simulink model "pure_pursuit"  (R2015b)
settings: Solver=FixedStepDiscrete  StartTime=0.0  StopTime=3  FixedStep=0.01  RelTol=1e-3
settings Model: Creator=castiel_liu  LastModifiedBy=castiel_liu

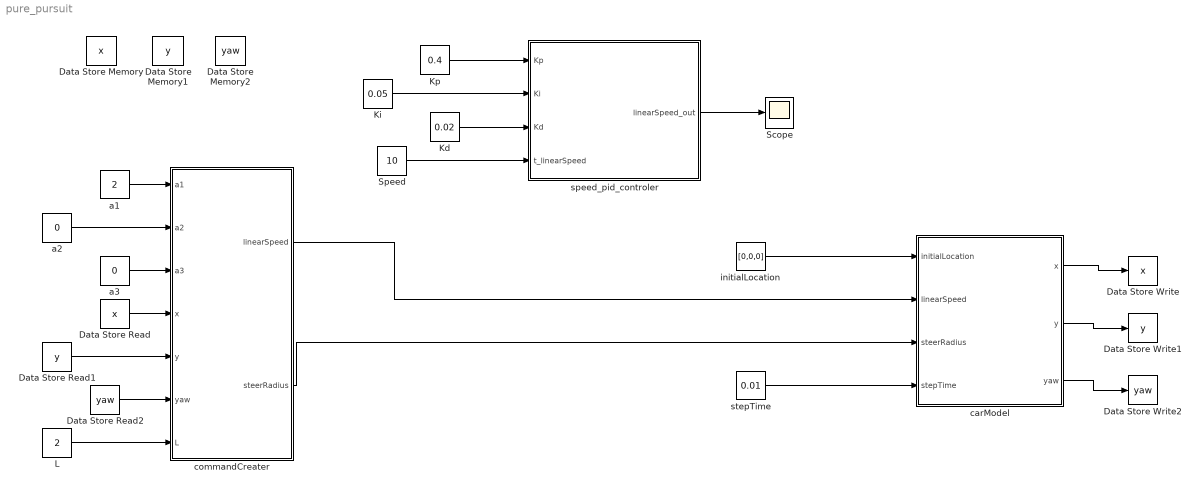
== system pure_pursuit ==
  Data Store Memory : DataStoreMemory  DataStoreName=x  ReadBeforeWriteMsg=warning  WriteAfterWriteMsg=warning  WriteAfterReadMsg=warning
  Data Store Memory1 : DataStoreMemory  DataStoreName=y  ReadBeforeWriteMsg=warning  WriteAfterWriteMsg=warning  WriteAfterReadMsg=warning
  Data Store Memory2 : DataStoreMemory  DataStoreName=yaw  ReadBeforeWriteMsg=warning  WriteAfterWriteMsg=warning  WriteAfterReadMsg=warning
  Data Store Read : DataStoreRead  DataStoreName=x
  Data Store Read1 : DataStoreRead  DataStoreName=y
  Data Store Read2 : DataStoreRead  DataStoreName=yaw
  Data Store Write : DataStoreWrite  DataStoreName=x
  Data Store Write1 : DataStoreWrite  DataStoreName=y
  Data Store Write2 : DataStoreWrite  DataStoreName=yaw
  Kd : Constant  Value=0.02
  Ki : Constant  Value=0.05
  Kp : Constant  Value=0.4
  L : Constant  Value=2
  Scope : Scope
  Speed : Constant  Value=10
  a1 : Constant  Value=2
  a2 : Constant  Value=0
  a3 : Constant  Value=0
  "carModel " : MATLAB Function  TreatAsAtomicUnit=on
  commandCreater : MATLAB Function  TreatAsAtomicUnit=on
  initialLocation : Constant  Value=[0,0,0]
  speed_pid_controler : MATLAB Function  TreatAsAtomicUnit=on
  stepTime : Constant  Value=0.01
  wires:
  stepTime/1 -> "carModel "/4(stepTime)
  commandCreater/1(linearSpeed) -> "carModel "/2(linearSpeed)
  commandCreater/2(steerRadius) -> "carModel "/3(steerRadius)
  L/1 -> commandCreater/7(L)
  "carModel "/2(y) -> Data Store Write1/1
  "carModel "/1(x) -> Data Store Write/1
  Data Store Read/1 -> commandCreater/4(x)
  Data Store Read1/1 -> commandCreater/5(y)
  Data Store Read2/1 -> commandCreater/6(yaw)
  "carModel "/3(yaw) -> Data Store Write2/1
  a2/1 -> commandCreater/2(a2)
  a3/1 -> commandCreater/3(a3)
  a1/1 -> commandCreater/1(a1)
  initialLocation/1 -> "carModel "/1(initialLocation)
  Kd/1 -> speed_pid_controler/3(Kd)
  Ki/1 -> speed_pid_controler/2(Ki)
  Kp/1 -> speed_pid_controler/1(Kp)
  speed_pid_controler/1(linearSpeed_out) -> Scope/1
  Speed/1 -> speed_pid_controler/4(t_linearSpeed)

== matlab function pure_pursuit/carModel  ==
  data: initialLocation input; linearSpeed input; x output; steerRadius input; y output; stepTime input; yaw output
function [x,y,yaw] = fcn(initialLocation,linearSpeed,steerRadius,stepTime)
%#
persistent x0;
persistent y0;
persistent theta0;
persistent first_time_flag;

if(isempty(x0))
    x0 = 0;
    y0 = 0;
    theta0 = 0.0;
    first_time_flag = 1;
end

fp = fopen('record.txt','a');
if(first_time_flag == 1)
    x=initialLocation(1);
    y=initialLocation(2);
    yaw = initialLocation(3);
    first_time_flag = 0;
else
    angularSpeed = linearSpeed / (steerRadius);

    theta = angularSpeed * stepTime;
    alpha = theta/2;
    if(alpha ~=0)
        rho = 2*steerRadius*sin(alpha); 
    else
        rho = linearSpeed * stepTime;
    end
    %旋转坐标变换矩阵
    convertMatrix = [cos(theta0),sin(theta0);-sin(theta0),cos(theta0)];

    temp = convertMatrix * [rho*cos(alpha),rho*sin(alpha)]'+[x0;y0];
    x = temp(1);
    y = temp(2);
    yaw = -( theta0+theta);
end

x0 = x;
y0 = y;
theta0 =-yaw;
    

fprintf(fp,'%f\t%f\n',x,y); 
%fprintf('%f\t%f\n',x,y);
fclose(fp);


end

== matlab function pure_pursuit/speed_pid_controler ==
  data: Kp input; Ki input; linearSpeed_out output; Kd input; t_linearSpeed input
function linearSpeed_out = fcn(Kp,Ki,Kd,t_linearSpeed)
persistent last_err
persistent last_last_err
persistent sigma_err
persistent last_val %上一次的值

if(isempty(last_err))
    last_err = 0;
    sigma_err = 0;
    last_val =0;
    last_last_err=0;
end 

err = t_linearSpeed - last_val;
sigma_err = sigma_err + err;
linearSpeed_out = Kp *err +Ki*sigma_err +Kd* (err-last_err);
%linearSpeed_out = Kp*(err-last_err) +Ki*err +Kd*(err-2*last_err+last_last_err);
last_last_err = last_err;
last_err = err;
last_val = linearSpeed_out;

fprintf('%f\t%f\t%f\n',err,linearSpeed_out,sigma_err);
end

== matlab function pure_pursuit/commandCreater ==
  data: a1 input; a2 input; a3 input; linearSpeed output; steerRadius output; x input; y input; yaw input; L input
function [linearSpeed,steerRadius] = fcn(a1,a2,a3,x,y,yaw,L)
persistent target_x;
persistent target_y;
if(isempty(target_x))
    target_x = 0;
end
% if(isempty(target_y))
%     target_y = 0;
% end


target_y = a1*target_x + a2*target_x^2 + a3*target_x^3;
%target_y = sin(target_x);
dis = (target_y-y)^2+(target_x-x)^2;
t_yaw = atan2(target_y-y,target_x-x);
if(dis < L*L)
    target_x = target_x +0.01;
    linearSpeed = 0;
    steerRadius = inf;
else
    linearSpeed = 2;
    steerRadius = -L/(2*sin(t_yaw-yaw));
    if(steerRadius >30) 
        steerRadius=inf;
    end
end

%fprintf('%f\t%f\t%f\t%f\t%f\t%f\t%f\n',t_yaw*180/pi,yaw*180/pi,steerRadius,linearSpeed, sqrt(dis),target_x,target_y);
    
end
